simulink model "sampleModel125"  (R2021b)
settings: Solver=VariableStepAuto  StartTime=0.0  StopTime=10.0  RelTol=1e-3
undefined symbols (not defined in the file or in its folder): DiscIntNeverNeededParam
libraries: simulink x7, slpidlib x2
settings Model: Creator=user  LastModifiedBy=user

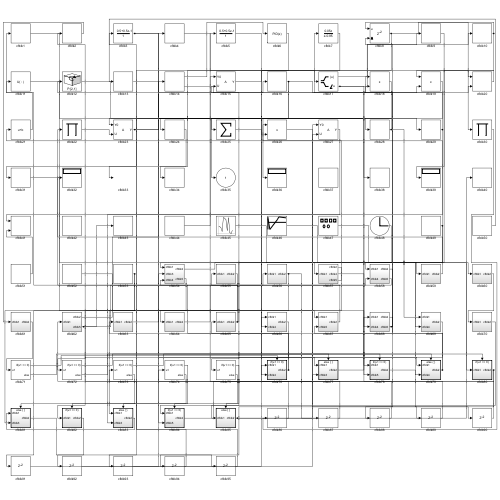
[thumbnail: Simulink's stored preview of the top-level diagram]
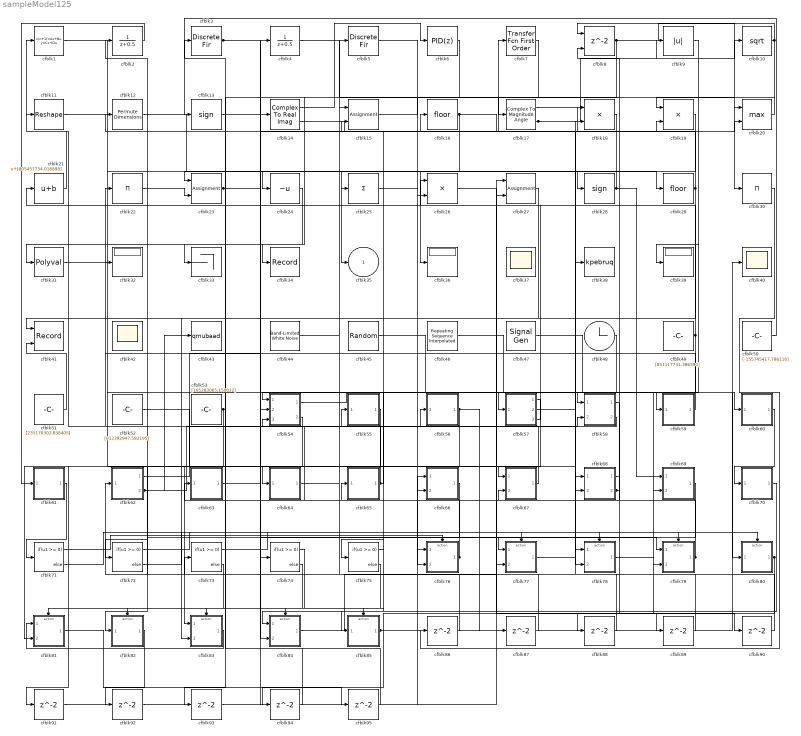
== system sampleModel125 ==
  cfblk1 : DiscreteStateSpace
  cfblk10 : Sqrt  SaturateOnIntegerOverflow=on
  cfblk11 : Reshape
  cfblk12 : PermuteDimensions
  cfblk13 : Signum
  cfblk14 : ComplexToRealImag
  cfblk15 : Assignment  DiagnosticForDimensions=Warning  IndexOptions=Index vector (dialog)  Indices=1  OutputSizes=1
  cfblk16 : Rounding
  cfblk17 : ComplexToMagnitudeAngle
  cfblk18 : Product
  cfblk19 : Product
  cfblk2 : DiscreteTransferFcn  SampleTime=1
  cfblk20 : MinMax  Function=max  Inputs=2
  cfblk21 : Bias  Bias=[805457734.016898]
  cfblk22 : Product  Inputs=*
  cfblk23 : Assignment  DiagnosticForDimensions=Warning  IndexOptions=Index vector (dialog)  Indices=1  OutputSizes=1
  cfblk24 : UnaryMinus
  cfblk25 : Sum  Inputs=+
  cfblk26 : Product  Inputs=**
  cfblk27 : Assignment  DiagnosticForDimensions=Warning  IndexOptions=Index vector (dialog)  Indices=1  OutputSizes=1
  cfblk28 : Signum
  cfblk29 : Rounding
  cfblk3 : DiscreteFir  SampleTime=1
  cfblk30 : Product  Inputs=*
  cfblk31 : Polyval  Coefs=[ +2.081618890e-019, -1.441693666e-014, +4.719686976e-010, -8.536869453e-006, +1.621573104e-001, -8.087801117e+001 ]
  cfblk32 : Display
  cfblk33 : Terminator
  cfblk34 : Record  FileSettingsInternal="{\"entries\":[{\"content\":{\"excelSettings\":{\"content\":{},\"type\":\"Streamout.ExcelSettings\"}},\"type\":\"Streamout.FileSettingStorage\",\"uuid\":\"10b3a829-3b43-40bf-bdec-2873be39b544\"}],\"packageUris\":[\"http://schema.mathworks.com/mf0/streamout_blocks/R2020a\"],\"version\":\"1.0\"}"  SignalsInternal="{\"entries\":[{\"content\":{\"signals\":[{\"content\":{\"blockPath\":[\"sampleModel125/cfblk34\"],\"channel\":[],\"dimensions\":[1],\"domain\":\"sampleModel125/cfblk34\",\"lineColor\":\"#4dbeee\",\"plots\":[1],\"port\":1,\"sid\":[\"\"],\"signalID\":4407,\"signalName\":\"cfblk6\"},\"type\":\"RecordBlkView.Signal\",\"uuid\":\"dde6bba3-9d79-403d-9fee-fe8c637f291d\"}]},\"type\":\"RecordBlkView.InputSignals\",\"uuid\":\"595af941-56f7-477e-9f25-0f9a9aec7386\"}],\"packageUris\":[\"http://schema.mathworks.com/mf0/streamout_blocks/R2020a\"],\"version\":\"1.0\"}"  VisualizationBindings="{\"sparklinesplugin\":{\"info\":[{\"bindingParametersList\":[],\"subplotID\":1}]}}"
  cfblk36 : Display
  cfblk37 : Scope
      settings: Floating=on
  cfblk38 : ToWorkspace  VariableName=kpebruq  SaveFormat=Timeseries  SampleTime=-1
  cfblk39 : Display
  cfblk4 : DiscreteTransferFcn  SampleTime=1
  cfblk40 : Scope
  cfblk41 : Record  FileSettingsInternal="{\"entries\":[{\"content\":{\"excelSettings\":{\"content\":{},\"type\":\"Streamout.ExcelSettings\"}},\"type\":\"Streamout.FileSettingStorage\",\"uuid\":\"c1591aa4-c251-4cb9-a9b5-7e1959374f39\"}],\"packageUris\":[\"http://schema.mathworks.com/mf0/streamout_blocks/R2020a\"],\"version\":\"1.0\"}"  Layout=[1 1]  SignalsInternal="{\"entries\":[{\"content\":{\"signals\":[{\"content\":{\"blockPath\":[\"sampleModel125/cfblk41\"],\"channel\":[],\"dimensions\":[1],\"domain\":\"sampleModel125/cfblk41\",\"lineColor\":\"#a2142f\",\"plots\":[1],\"port\":1,\"sid\":[\"\"],\"signalID\":4411,\"signalName\":\"cfblk27\"},\"type\":\"RecordBlkView.Signal\",\"uuid\":\"4e167d94-f253-4071-9bb9-3a192c00a069\"},{\"content\":{\"blockPath\":[\"sampleModel125/cfblk41\"],\"channel\":[],\"dimensions\":[1],\"domain\":\"sampleModel125/cfblk41\",\"lineColor\":\"#139fff\",\"plots\":[1],\"port\":2,\"sid\":[\"\"],\"signalID\":4415,\"signalName\":\"cfblk51\"},\"type\":\"RecordBlkView.Signal\",\"uuid\":\"893185ae-1f6e-475b-a7d2-7c6d7e90e1fb\"}]},\"type\":\"RecordBlkView.InputSignals\",\"uuid\":\"ca8d18b8-456d-47c3-8407-3c84aebed2dd\"}],\"packageUris\":[\"http://schema.mathworks.com/mf0/streamout_blocks/R2020a\"],\"version\":\"1.0\"}"  VisualizationBindings="{\"xyplotplugin\":{\"info\":[{\"series\":[{\"bindingParametersList\":[{\"parameter\":\"X-Axis\",\"signalID\":4411,\"signalName\":\"cfblk27\"},{\"parameter\":\"Y-Axis\",\"signalID\":4415,\"signalName\":\"cfblk51\"}],\"seriesID\":13289}],\"subplotID\":1}]}}"  CompatibilityTag=XY
  cfblk42 : Scope
      settings: Floating=on
  cfblk43 : ToWorkspace  VariableName=qmubaad  SaveFormat=Timeseries  SampleTime=-1
  cfblk44 : simulink/Sources/Band-Limited White Noise  Cov=[5500056983.658573]  Ts=0.1  seed=[7259056382.000000]
  cfblk45 : RandomNumber  Mean=[-77643.430435]  Variance=[89785.458999]  Seed=[977465673.000000]  SampleTime=0.1
  cfblk46 : simulink/Sources/Repeating Sequence Interpolated  OutValues=[472862827.691020, -784261342.919639, 330374343.282986, 653758558.924161, 535953124.720396]  TimeValues=[0 0.1 0.5 0.6 1].'  LookUpMeth=Use Input Above  tsamp=0.01  OutMin=[]  OutMax=[]  OutDataTypeStr=double  OutputDataTypeScalingMode=double  OutDataType=fixdt(0,8)  OutScaling=2^-10
  cfblk47 : SignalGenerator  Amplitude=[910429593.160431]
  cfblk48 : Clock
  cfblk49 : Constant  Value=[851117741.386390]  SampleTime=1
  cfblk5 : DiscreteFir  SampleTime=1
  cfblk50 : Constant  Value=[-155745417.798116]  SampleTime=1
  cfblk51 : Constant  Value=[235170302.838405]  SampleTime=1
  cfblk52 : Constant  Value=[812392947.582195]  SampleTime=1
  cfblk53 : Constant  Value=[165283065.150022]  SampleTime=1
  cfblk54 : Subsystem
  cfblk55 : Subsystem
  cfblk56 : Subsystem
  cfblk57 : Subsystem
  cfblk58 : Subsystem
  cfblk59 : Subsystem
  cfblk6 : slpidlib/PID Controller  Controller=PID  Form=Parallel  TimeDomain=Discrete-time  UseExternalTs=off  SampleTime=1  IntegratorMethod=Forward Euler  FilterMethod=Forward Euler  ControllerParametersSource=internal  P=1  I=1  D=0  UseFilter=on  N=100  TunerSelectOption=Transfer Function Based (PID Tuner App)  InitialConditionSource=internal  InitialConditionForIntegrator=0  InitialConditionForFilter=0  DifferentiatorICPrevScaledInput=0  ExternalReset=none  TrackingMode=off  Kt=1  LimitOutput=off  SatLimitsSource=internal  UpperSaturationLimit=inf  LowerSaturationLimit=-inf  LinearizeAsGain=off  AntiWindupMode=none  Kb=1  POutMin=[]  POutMax=[]  IOutMin=[]  IOutMax=[]  DOutMin=[]  DOutMax=[]  NOutMin=[]  NOutMax=[]  SumOutMin=[]  SumOutMax=[]  SaturationOutMin=[]  SaturationOutMax=[]  PParamMin=[]  PParamMax=[]  IParamMin=[]  IParamMax=[]  DParamMin=[]  DParamMax=[]  NParamMin=[]  NParamMax=[]  KbParamMin=[]  KbParamMax=[]  KtParamMin=[]  KtParamMax=[]  KbOutMin=[]  KbOutMax=[]  KtOutMin=[]  KtOutMax=[]  IntegratorOutMin=[]  IntegratorOutMax=[]  FilterOutMin=[]  FilterOutMax=[]  SumI1OutMin=[]  SumI1OutMax=[]  SumI2OutMin=[]  SumI2OutMax=[]  SumI3OutMin=[]  SumI3OutMax=[]  SumI4OutMin=[]  SumI4OutMax=[]  SumDOutMin=[]  SumDOutMax=[]  DifferentiatorOutMin=[]  DifferentiatorOutMax=[]  FilterDiffOutCoefMin=[]  FilterDiffOutCoefMax=[]  ReciprocalOutMin=[]  ReciprocalOutMax=[]  SumDenOutMin=[]  SumDenOutMax=[]  SumNumOutMin=[]  SumNumOutMax=[]  DivideOutMin=[]  DivideOutMax=[]  UdiffTsProdOutMin=[]  UdiffTsProdOutMax=[]  NTsProdOutMin=[]  NTsProdOutMax=[]  UintegralTsProdOutMin=[]  UintegralTsProdOutMax=[]  UngainTsProdOutMin=[]  UngainTsProdOutMax=[]  IntegratorContinuousStateAttributes=''  IntegratorStateMustResolveToSignalObject=off  IntegratorRTWStateStorageClass=Auto  FilterContinuousStateAttributes=''  FilterStateMustResolveToSignalObject=off  FilterRTWStateStorageClass=Auto  ParallelPVariant=InternalParameters  IdealPVariant=Disabled  IVariant=InternalParameters  DVariant=InternalParameters  IntegratorVariant=Discrete  SatVariant=Disabled  AWVariant=Passthrough  PCopyVariant=Disabled  TRVariant=Disabled  FdbkBlocksVariant=Forward  IdealPFdbkVariant=Disabled  SatFdbkVariant=Disabled  DerivativeFilterVariant=ForwardEulerFilter  NVariant=InternalParameters  NCopyVariant=Disabled  FilterICVariant=InternalICsFilter  IntegratorICVariant=InternalICs  ExternalResetVariant=Disabled  TRSumVariant=Passthrough  SumFdbkVariant=Disabled  SumVariant=Sum_PID  TsampFilterVariant=InternalTs  TsampNgainVariant=Passthrough  TsampIntegralVariant=Passthrough  ExternalSaturationOutDataTypeStr=Inherit: Same as second input
  cfblk60 : Subsystem
  cfblk61 : Subsystem
  cfblk62 : Subsystem
  cfblk63 : Subsystem
  cfblk64 : Subsystem
  cfblk65 : Subsystem
  cfblk66 : Subsystem
  cfblk67 : Subsystem
  cfblk68 : Subsystem
  cfblk69 : Subsystem
  cfblk7 : simulink/Discrete/Transfer Fcn First Order  PoleZ=0.95  ICPrevOutput=0.0  DoSatur=off
  cfblk70 : Subsystem
  cfblk{71..75} (5 alike) : If  IfExpression=u1 >= 0  SampleTime=1
  cfblk76 : Subsystem  TreatAsAtomicUnit=on
  cfblk77 : Subsystem  TreatAsAtomicUnit=on
  cfblk78 : Subsystem  TreatAsAtomicUnit=on
  cfblk79 : Subsystem  TreatAsAtomicUnit=on
  cfblk8 : Delay  ShowEnablePort=on  SampleTime=1
      settings: InputPortMap=u0,e6
  cfblk80 : Subsystem  TreatAsAtomicUnit=on
  cfblk81 : Subsystem  TreatAsAtomicUnit=on
  cfblk82 : Subsystem  TreatAsAtomicUnit=on
  cfblk83 : Subsystem  TreatAsAtomicUnit=on
  cfblk84 : Subsystem  TreatAsAtomicUnit=on
  cfblk85 : Subsystem  TreatAsAtomicUnit=on
  cfblk{86..95} (10 alike) : Delay  SampleTime=1
  cfblk9 : Abs
  cfblk35 : Outport
  wires:
  cfblk60/1(cfblk2) -> cfblk70/1(cfblk1)
  cfblk19/1 -> cfblk23/1
  cfblk9/1 -> cfblk54/1(cfblk1)
  cfblk1/1 -> cfblk67/1(cfblk1)
  cfblk16/1 -> cfblk20/2, cfblk26/2, cfblk93/1
  cfblk80/1(cfblk2) -> cfblk62/1(cfblk1), cfblk94/1
  cfblk55/1(cfblk2) -> cfblk72/1
  cfblk27/1 -> cfblk41/1
  cfblk25/1 -> cfblk66/2(cfblk4)
  cfblk29/1 -> cfblk7/1, cfblk83/2(cfblk3)
  cfblk76/1(cfblk2) -> cfblk65/1(cfblk1), cfblk54/3(cfblk4)
  cfblk59/1(cfblk2) -> cfblk22/1
  cfblk53/1 -> cfblk83/1(cfblk1), cfblk81/2(cfblk3)
  cfblk21/1 -> cfblk1/1
  cfblk24/1 -> cfblk31/1
  cfblk70/1(cfblk2) -> cfblk84/1(cfblk1)
  cfblk28/1 -> cfblk24/1, cfblk69/1(cfblk1)
  cfblk56/1(cfblk2) -> cfblk84/2(cfblk5), cfblk87/1
  cfblk11/1 -> cfblk36/1
  cfblk44/1 -> cfblk5/1
  cfblk63/1(cfblk2) -> cfblk4/1
  cfblk49/1 -> cfblk58/1(cfblk1), cfblk8/2, cfblk69/2(cfblk4)
  cfblk64/1(cfblk2) -> cfblk56/1(cfblk1)
  cfblk14/1 -> cfblk6/1
  cfblk62/1(cfblk2) -> cfblk14/1
  cfblk6/1 -> cfblk34/1
  cfblk58/1(cfblk2) -> cfblk67/2(cfblk5)
  cfblk31/1 -> cfblk60/1(cfblk1)
  cfblk13/1 -> cfblk29/1
  cfblk23/1 -> cfblk28/1, cfblk18/2
  cfblk67/1(cfblk2) -> cfblk32/1
  cfblk8/1 -> cfblk30/1, cfblk33/1
  cfblk65/1(cfblk2) -> cfblk11/1, cfblk15/2
  cfblk58/2(cfblk5) -> cfblk55/1(cfblk1)
  cfblk7/1 -> cfblk76/2(cfblk4)
  cfblk62/2(cfblk5) -> cfblk58/2(cfblk4), cfblk43/1
  cfblk47/1 -> cfblk59/1(cfblk1)
  cfblk10/1 -> cfblk39/1, cfblk8/1
  cfblk18/1 -> cfblk35/1
  cfblk5/1 -> cfblk77/1(cfblk1)
  cfblk20/1 -> cfblk19/1
  cfblk12/1 -> cfblk78/1(cfblk1)
  cfblk45/1 -> cfblk80/1(cfblk1)
  cfblk79/1(cfblk2) -> cfblk63/1(cfblk1), cfblk18/1
  cfblk68/2(cfblk5) -> cfblk26/1, cfblk12/1
  cfblk57/1(cfblk2) -> cfblk64/1(cfblk1)
  cfblk85/1(cfblk2) -> cfblk27/1, cfblk40/1
  cfblk2/1 -> cfblk61/1(cfblk1)
  cfblk17/1 -> cfblk10/1
  cfblk66/1(cfblk2) -> cfblk82/1(cfblk1)
  cfblk22/1 -> cfblk23/2
  cfblk48/1 -> cfblk75/1
  cfblk61/1(cfblk2) -> cfblk71/1
  cfblk17/2 -> cfblk38/1, cfblk9/1
  cfblk84/1(cfblk2) -> cfblk27/2
  cfblk69/1(cfblk2) -> cfblk85/1(cfblk1)
  cfblk83/1(cfblk2) -> cfblk81/1(cfblk1)
  cfblk3/1 -> cfblk79/1(cfblk1), cfblk25/1
  cfblk14/2 -> cfblk16/1
  cfblk50/1 -> cfblk13/1
  cfblk46/1 -> cfblk79/2(cfblk4)
  cfblk54/1(cfblk2) -> cfblk57/1(cfblk1)
  cfblk51/1 -> cfblk41/2
  cfblk57/2(cfblk4) -> cfblk68/2(cfblk4)
  cfblk15/1 -> cfblk17/1
  cfblk52/1 -> cfblk78/2(cfblk5)
  cfblk4/1 -> cfblk20/1
  cfblk77/1(cfblk2) -> cfblk19/2
  cfblk57/3(cfblk5) -> cfblk21/1
  cfblk71/1 -> cfblk76/Action
  cfblk71/2 -> cfblk77/Action
  cfblk72/1 -> cfblk78/Action
  cfblk72/2 -> cfblk79/Action
  cfblk73/1 -> cfblk80/Action
  cfblk73/2 -> cfblk81/Action
  cfblk74/1 -> cfblk82/Action
  cfblk74/2 -> cfblk83/Action
  cfblk75/1 -> cfblk84/Action
  cfblk75/2 -> cfblk85/Action
  cfblk30/1 -> cfblk86/1
  cfblk86/1 -> cfblk76/1(cfblk1)
  cfblk87/1 -> cfblk15/1
  cfblk68/1(cfblk2) -> cfblk88/1
  cfblk88/1 -> cfblk54/2(cfblk3)
  cfblk26/1 -> cfblk89/1
  cfblk89/1 -> cfblk2/1
  cfblk78/1(cfblk2) -> cfblk90/1
  cfblk90/1 -> cfblk68/1(cfblk1)
  cfblk54/2(cfblk5) -> cfblk91/1
  cfblk91/1 -> cfblk77/2(cfblk3)
  cfblk82/1(cfblk2) -> cfblk92/1
  cfblk92/1 -> cfblk74/1
  cfblk93/1 -> cfblk66/1(cfblk1)
  cfblk94/1 -> cfblk3/1
  cfblk81/1(cfblk2) -> cfblk95/1
  cfblk95/1 -> cfblk73/1

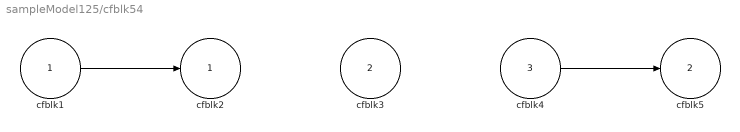
== system sampleModel125/cfblk54 ==
  cfblk1 : Inport
  cfblk3 : Inport  Port=2
  cfblk4 : Inport  Port=3
  cfblk2 : Outport
  cfblk5 : Outport  Port=2
  wires:
  cfblk1/1 -> cfblk2/1
  cfblk4/1 -> cfblk5/1

== system sampleModel125/cfblk55 ==
  cfblk1 : Inport
  cfblk3 : Trigonometry
  cfblk4 : Constant  Value=[-689189918.602560]  SampleTime=1
  cfblk2 : Outport
  wires:
  cfblk4/1 -> cfblk3/1
  cfblk3/1 -> cfblk2/1

== system sampleModel125/cfblk56 ==
  cfblk1 : Inport
  cfblk3 : Gain  Gain=[-567529221.221164]
  cfblk2 : Outport
  wires:
  cfblk1/1 -> cfblk3/1
  cfblk3/1 -> cfblk2/1

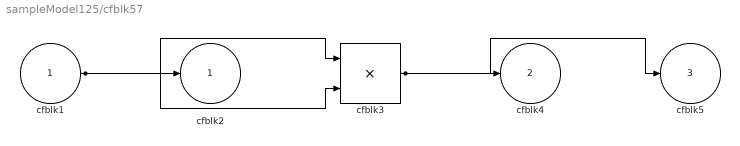
== system sampleModel125/cfblk57 ==
  cfblk1 : Inport
  cfblk3 : Product
  cfblk2 : Outport
  cfblk4 : Outport  Port=2
  cfblk5 : Outport  Port=3
  wires:
  cfblk3/1 -> cfblk5/1, cfblk4/1
  cfblk1/1 -> cfblk2/1, cfblk3/1, cfblk3/2

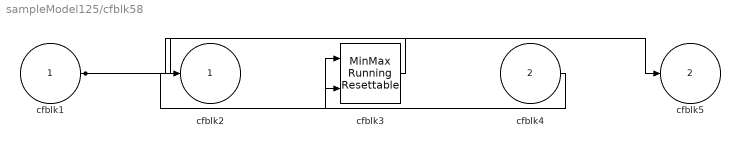
== system sampleModel125/cfblk58 ==
  cfblk1 : Inport
  cfblk4 : Inport  Port=2
  cfblk3 : simulink/Math Operations/MinMax Running Resettable  Function=min  vinit=0.0
  cfblk2 : Outport
  cfblk5 : Outport  Port=2
  wires:
  cfblk1/1 -> cfblk5/1, cfblk3/2
  cfblk4/1 -> cfblk3/1
  cfblk3/1 -> cfblk2/1

== system sampleModel125/cfblk59 ==
  cfblk1 : Inport
  cfblk3 : DiscreteTransferFcn  SampleTime=1
  cfblk2 : Outport
  wires:
  cfblk1/1 -> cfblk3/1
  cfblk3/1 -> cfblk2/1

== system sampleModel125/cfblk60 ==
  cfblk1 : Inport
  cfblk3 : DiscreteIntegrator  ICPrevOutput=DiscIntNeverNeededParam  ICPrevScaledInput=DiscIntNeverNeededParam
  cfblk4 : Squeeze
  cfblk2 : Outport
  wires:
  cfblk1/1 -> cfblk3/1
  cfblk3/1 -> cfblk4/1
  cfblk4/1 -> cfblk2/1

== system sampleModel125/cfblk61 ==
  cfblk1 : Inport
  cfblk3 : Product  Inputs=**
  cfblk2 : Outport
  wires:
  cfblk1/1 -> cfblk3/1, cfblk3/2
  cfblk3/1 -> cfblk2/1

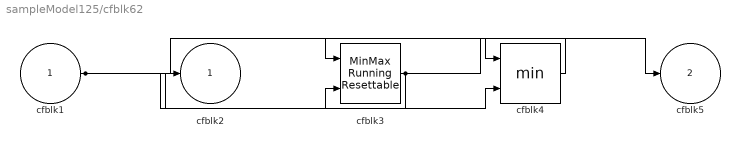
== system sampleModel125/cfblk62 ==
  cfblk1 : Inport
  cfblk3 : simulink/Math Operations/MinMax Running Resettable  Function=min  vinit=0.0
  cfblk4 : MinMax  Inputs=2
  cfblk2 : Outport
  cfblk5 : Outport  Port=2
  wires:
  cfblk1/1 -> cfblk4/1, cfblk3/2, cfblk4/2
  cfblk3/1 -> cfblk2/1, cfblk5/1
  cfblk4/1 -> cfblk3/1

== system sampleModel125/cfblk63 ==
  cfblk1 : Inport
  cfblk3 : Reshape
  cfblk4 : Constant  Value=[804097030.204221]  SampleTime=1
  cfblk2 : Outport
  wires:
  cfblk4/1 -> cfblk2/1
  cfblk1/1 -> cfblk3/1

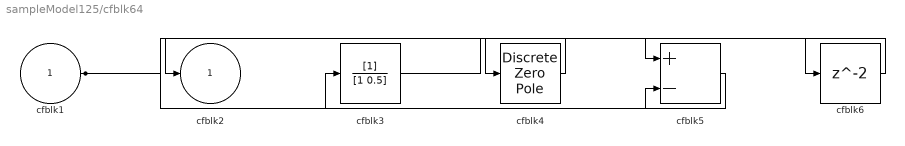
== system sampleModel125/cfblk64 ==
  cfblk1 : Inport
  cfblk3 : DiscreteFilter  SampleTime=1
  cfblk4 : DiscreteZeroPole  Poles=[0 0.5]  Gain=1
  cfblk5 : Sum  Inputs=+-
  cfblk6 : Delay  SampleTime=1
  cfblk2 : Outport
  wires:
  cfblk4/1 -> cfblk2/1
  cfblk5/1 -> cfblk3/1
  cfblk1/1 -> cfblk4/1, cfblk5/2
  cfblk3/1 -> cfblk6/1
  cfblk6/1 -> cfblk5/1

== system sampleModel125/cfblk65 ==
  cfblk1 : Inport
  cfblk3 : Sqrt  SaturateOnIntegerOverflow=on
  cfblk2 : Outport
  wires:
  cfblk1/1 -> cfblk3/1
  cfblk3/1 -> cfblk2/1

== system sampleModel125/cfblk66 ==
  cfblk1 : Inport
  cfblk4 : Inport  Port=2
  cfblk3 : simulink/Discrete/Transfer Fcn Lead or Lag  PoleZ=0.95  ZeroZ=0.75  ICPrevOutput=0.0  ICPrevInput=0.0  DoSatur=off
      settings: SourceProductBaseCode=SL
  cfblk2 : Outport
  wires:
  cfblk3/1 -> cfblk2/1
  cfblk4/1 -> cfblk3/1

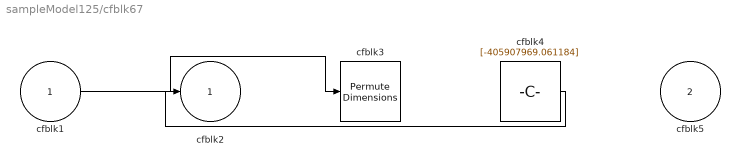
== system sampleModel125/cfblk67 ==
  cfblk1 : Inport
  cfblk5 : Inport  Port=2
  cfblk3 : PermuteDimensions
  cfblk4 : Constant  Value=[-405907969.061184]  SampleTime=1
  cfblk2 : Outport
  wires:
  cfblk1/1 -> cfblk3/1
  cfblk4/1 -> cfblk2/1

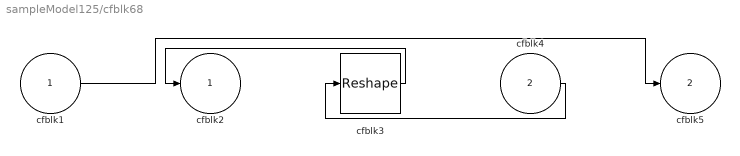
== system sampleModel125/cfblk68 ==
  cfblk1 : Inport
  cfblk4 : Inport  Port=2
  cfblk3 : Reshape
  cfblk2 : Outport
  cfblk5 : Outport  Port=2
  wires:
  cfblk3/1 -> cfblk2/1
  cfblk4/1 -> cfblk3/1
  cfblk1/1 -> cfblk5/1

== system sampleModel125/cfblk69 ==
  cfblk1 : Inport
  cfblk4 : Inport  Port=2
  cfblk3 : simulink/Discrete/Difference  ICPrevInput=0.0  OutMin=[]  OutMax=[]  OutDataTypeStr=Inherit: Inherit via back propagation  OutDataType=fixdt(1, 16)  OutScaling=2^-10  DoSatur=off
  cfblk2 : Outport
  wires:
  cfblk4/1 -> cfblk2/1
  cfblk1/1 -> cfblk3/1

== system sampleModel125/cfblk70 ==
  cfblk1 : Inport
  cfblk3 : Product  Inputs=**
  cfblk2 : Outport
  wires:
  cfblk3/1 -> cfblk2/1
  cfblk1/1 -> cfblk3/1, cfblk3/2

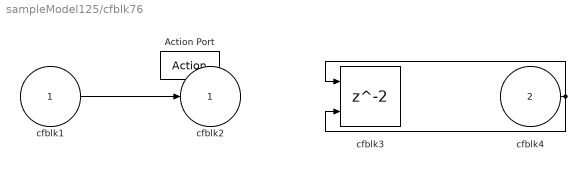
== system sampleModel125/cfblk76 ==
  cfblk1 : Inport
  cfblk4 : Inport  Port=2
  Action Port : ActionPort  ActionPortLabel=if(u1 >= 0)
  cfblk3 : Delay  ShowEnablePort=on
      settings: InputPortMap=u0,e6
  cfblk2 : Outport
  wires:
  cfblk1/1 -> cfblk2/1
  cfblk4/1 -> cfblk3/1, cfblk3/2

== system sampleModel125/cfblk77 ==
  cfblk1 : Inport
  cfblk3 : Inport  Port=2
  Action Port : ActionPort  ActionPortLabel=else
  cfblk2 : Outport
  wires:
  cfblk1/1 -> cfblk2/1

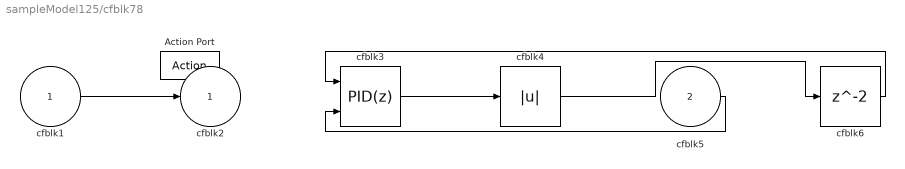
== system sampleModel125/cfblk78 ==
  cfblk1 : Inport
  cfblk5 : Inport  Port=2
  Action Port : ActionPort  ActionPortLabel=if(u1 >= 0)
  cfblk3 : slpidlib/PID Controller (2DOF)  Controller=PID  Form=Parallel  TimeDomain=Discrete-time  UseExternalTs=off  SampleTime=-1  IntegratorMethod=Forward Euler  FilterMethod=Forward Euler  ControllerParametersSource=internal  P=1  I=1  D=0  UseFilter=on  N=100  b=1  c=1  TunerSelectOption=Transfer Function Based (PID Tuner App)  InitialConditionSource=internal  InitialConditionForIntegrator=0  InitialConditionForFilter=0  DifferentiatorICPrevScaledInput=0  ExternalReset=none  TrackingMode=off  Kt=1  LimitOutput=off  SatLimitsSource=internal  UpperSaturationLimit=inf  LowerSaturationLimit=-inf  LinearizeAsGain=off  AntiWindupMode=none  Kb=1  POutMin=[]  POutMax=[]  IOutMin=[]  IOutMax=[]  DOutMin=[]  DOutMax=[]  NOutMin=[]  NOutMax=[]  bOutMin=[]  bOutMax=[]  cOutMin=[]  cOutMax=[]  SumOutMin=[]  SumOutMax=[]  SaturationOutMin=[]  SaturationOutMax=[]  PParamMin=[]  PParamMax=[]  IParamMin=[]  IParamMax=[]  DParamMin=[]  DParamMax=[]  NParamMin=[]  NParamMax=[]  bParamMin=[]  bParamMax=[]  cParamMin=[]  cParamMax=[]  KbParamMin=[]  KbParamMax=[]  KtParamMin=[]  KtParamMax=[]  KbOutMin=[]  KbOutMax=[]  KtOutMin=[]  KtOutMax=[]  IntegratorOutMin=[]  IntegratorOutMax=[]  FilterOutMin=[]  FilterOutMax=[]  SumI1OutMin=[]  SumI1OutMax=[]  SumI2OutMin=[]  SumI2OutMax=[]  SumI3OutMin=[]  SumI3OutMax=[]  SumI4OutMin=[]  SumI4OutMax=[]  SumDOutMin=[]  SumDOutMax=[]  Sum1OutMin=[]  Sum1OutMax=[]  Sum2OutMin=[]  Sum2OutMax=[]  Sum3OutMin=[]  Sum3OutMax=[]  DifferentiatorOutMin=[]  DifferentiatorOutMax=[]  FilterDiffOutCoefMin=[]  FilterDiffOutCoefMax=[]  ReciprocalOutMin=[]  ReciprocalOutMax=[]  SumDenOutMin=[]  SumDenOutMax=[]  SumNumOutMin=[]  SumNumOutMax=[]  DivideOutMin=[]  DivideOutMax=[]  UdiffTsProdOutMin=[]  UdiffTsProdOutMax=[]  NTsProdOutMin=[]  NTsProdOutMax=[]  UintegralTsProdOutMin=[]  UintegralTsProdOutMax=[]  UngainTsProdOutMin=[]  UngainTsProdOutMax=[]  IntegratorContinuousStateAttributes=''  IntegratorStateMustResolveToSignalObject=off  IntegratorRTWStateStorageClass=Auto  FilterContinuousStateAttributes=''  FilterStateMustResolveToSignalObject=off  FilterRTWStateStorageClass=Auto  ParallelPVariant=InternalParameters  IdealPVariant=Disabled  IVariant=InternalParameters  DVariant=InternalParameters  bVariant=InternalParameters  cVariant=InternalParameters  IntegratorVariant=Discrete  SatVariant=Disabled  AWVariant=Passthrough  PCopyVariant=Disabled  TRVariant=Disabled  FdbkBlocksVariant=Forward  IdealPFdbkVariant=Disabled  SatFdbkVariant=Disabled  DerivativeFilterVariant=ForwardEulerFilter  NVariant=InternalParameters  NCopyVariant=Disabled  FilterICVariant=InternalICsFilter  IntegratorICVariant=InternalICs  ExternalResetVariant=Disabled  TRSumVariant=Passthrough  SumFdbkVariant=Disabled  SumVariant=Sum_PID  TsampFilterVariant=InternalTs  TsampNgainVariant=Passthrough  TsampIntegralVariant=Passthrough  ExternalSaturationOutDataTypeStr=Inherit: Same as second input
      settings: SourceProductBaseCode=SL
  cfblk4 : Abs
  cfblk6 : Delay
  cfblk2 : Outport
  wires:
  cfblk1/1 -> cfblk2/1
  cfblk5/1 -> cfblk3/2
  cfblk3/1 -> cfblk4/1
  cfblk4/1 -> cfblk6/1
  cfblk6/1 -> cfblk3/1

== system sampleModel125/cfblk79 ==
  cfblk1 : Inport
  cfblk4 : Inport  Port=2
  Action Port : ActionPort  ActionPortLabel=else
  cfblk3 : DiscreteTransferFcn
  cfblk2 : Outport
  wires:
  cfblk1/1 -> cfblk3/1
  cfblk4/1 -> cfblk2/1

== system sampleModel125/cfblk80 ==
  cfblk1 : Inport
  Action Port : ActionPort  ActionPortLabel=if(u1 >= 0)
  cfblk3 : Polyval  Coefs=[ +2.081618890e-019, -1.441693666e-014, +4.719686976e-010, -8.536869453e-006, +1.621573104e-001, -8.087801117e+001 ]
  cfblk2 : Outport
  wires:
  cfblk3/1 -> cfblk2/1
  cfblk1/1 -> cfblk3/1

== system sampleModel125/cfblk81 ==
  cfblk1 : Inport
  cfblk3 : Inport  Port=2
  Action Port : ActionPort  ActionPortLabel=else
  cfblk2 : Outport
  wires:
  cfblk3/1 -> cfblk2/1

== system sampleModel125/cfblk82 ==
  cfblk1 : Inport
  Action Port : ActionPort  ActionPortLabel=if(u1 >= 0)
  cfblk3 : Trigonometry
  cfblk2 : Outport
  wires:
  cfblk1/1 -> cfblk3/1
  cfblk3/1 -> cfblk2/1

== system sampleModel125/cfblk83 ==
  cfblk1 : Inport
  cfblk3 : Inport  Port=2
  Action Port : ActionPort  ActionPortLabel=else
  cfblk2 : Outport
  wires:
  cfblk1/1 -> cfblk2/1

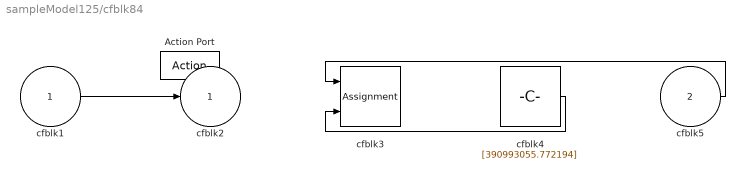
== system sampleModel125/cfblk84 ==
  cfblk1 : Inport
  cfblk5 : Inport  Port=2
  Action Port : ActionPort  ActionPortLabel=if(u1 >= 0)
  cfblk3 : Assignment  DiagnosticForDimensions=Warning  IndexOptions=Index vector (dialog)  Indices=1  OutputSizes=1
  cfblk4 : Constant  Value=[390993055.772194]  SampleTime=1
  cfblk2 : Outport
  wires:
  cfblk1/1 -> cfblk2/1
  cfblk5/1 -> cfblk3/1
  cfblk4/1 -> cfblk3/2

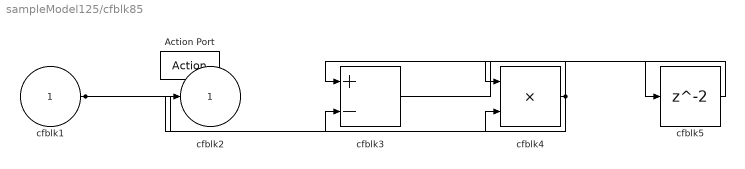
== system sampleModel125/cfblk85 ==
  cfblk1 : Inport
  Action Port : ActionPort  ActionPortLabel=else
  cfblk3 : Sum  Inputs=+-
  cfblk4 : Product  Inputs=**
  cfblk5 : Delay
  cfblk2 : Outport
  wires:
  cfblk1/1 -> cfblk4/2, cfblk3/2
  cfblk4/1 -> cfblk3/1, cfblk2/1
  cfblk3/1 -> cfblk5/1
  cfblk5/1 -> cfblk4/1
